simulink model "NonLinearModelPID_DT"  (R2018b)
settings: Solver=VariableStepAuto  StartTime=0.0  StopTime=50  RelTol=1e-3
undefined symbols (not defined in the file): DiscIntNeverNeededParam, Gxd_A_obs, Gxd_B_obs, Gxd_C_obs, Gyawd_A_obs, Gyawd_B_obs, Gyawd_C_obs, Gyd_A_obs, Gyd_B_obs, Gyd_C_obs, Gzd_A_obs, Gzd_B_obs, Gzd_C_obs, K0_X, K0_Y, K0_yaw, K0_Z, K_X, K_Y, K_yaw, K_Z, KGe_X, KGe_Y, KGe_yaw, KGe_Z, t_samp
libraries: simulink x5
settings Model: Creator=Henrique  LastModifiedBy=Henrique

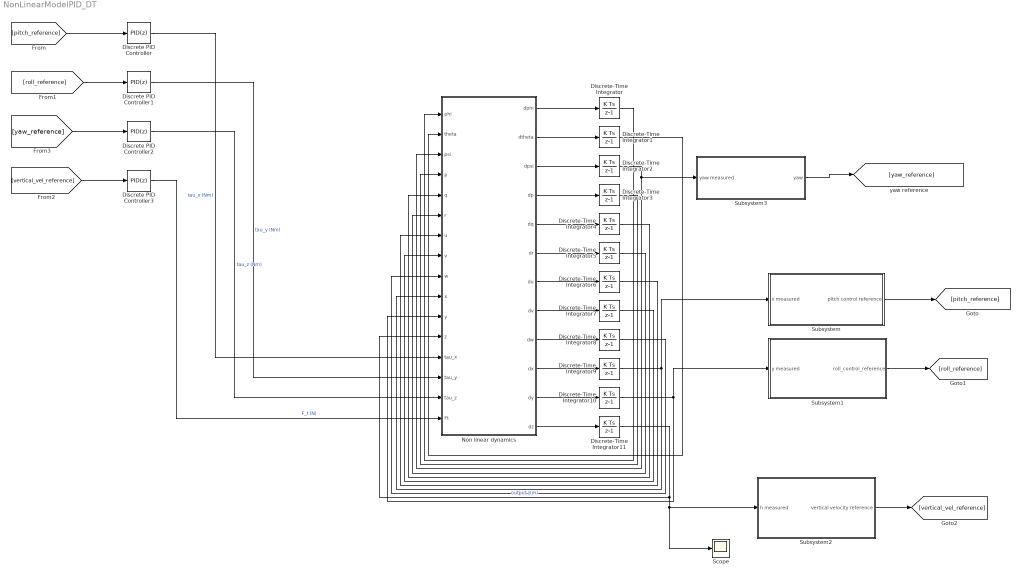
== system NonLinearModelPID_DT ==
  Discrete PID Controller : simulink/Continuous/PID Controller  Controller=PID  Form=Parallel  TimeDomain=Discrete-time  SampleTime=-1  IntegratorMethod=Forward Euler  FilterMethod=Forward Euler  ControllerParametersSource=internal  P=-0.0333564660904056  I=-0.00367562518786493  D=0.0674784843331279  UseFilter=on  N=0.484796452160315  TunerSelectOption=Transfer Function Based (PID Tuner App)  InitialConditionSource=internal  InitialConditionForIntegrator=0  InitialConditionForFilter=0  DifferentiatorICPrevScaledInput=0  ExternalReset=none  TrackingMode=off  Kt=1  LimitOutput=off  UpperSaturationLimit=inf  LowerSaturationLimit=-inf  LinearizeAsGain=off  AntiWindupMode=none  Kb=1  POutMin=[]  POutMax=[]  IOutMin=[]  IOutMax=[]  DOutMin=[]  DOutMax=[]  NOutMin=[]  NOutMax=[]  SumOutMin=[]  SumOutMax=[]  SaturationOutMin=[]  SaturationOutMax=[]  PParamMin=[]  PParamMax=[]  IParamMin=[]  IParamMax=[]  DParamMin=[]  DParamMax=[]  NParamMin=[]  NParamMax=[]  KbParamMin=[]  KbParamMax=[]  KtParamMin=[]  KtParamMax=[]  KbOutMin=[]  KbOutMax=[]  KtOutMin=[]  KtOutMax=[]  IntegratorOutMin=[]  IntegratorOutMax=[]  FilterOutMin=[]  FilterOutMax=[]  SumI1OutMin=[]  SumI1OutMax=[]  SumI2OutMin=[]  SumI2OutMax=[]  SumI3OutMin=[]  SumI3OutMax=[]  SumI4OutMin=[]  SumI4OutMax=[]  SumDOutMin=[]  SumDOutMax=[]  DifferentiatorOutMin=[]  DifferentiatorOutMax=[]  FilterDiffOutCoefMin=[]  FilterDiffOutCoefMax=[]  ReciprocalOutMin=[]  ReciprocalOutMax=[]  SumDenOutMin=[]  SumDenOutMax=[]  SumNumOutMin=[]  SumNumOutMax=[]  DivideOutMin=[]  DivideOutMax=[]  IntegratorContinuousStateAttributes=''  IntegratorStateMustResolveToSignalObject=off  IntegratorRTWStateStorageClass=Auto  FilterContinuousStateAttributes=''  FilterStateMustResolveToSignalObject=off  FilterRTWStateStorageClass=Auto  ParallelPVariant=InternalParameters  IdealPVariant=Disabled  IVariant=InternalParameters  DVariant=InternalParameters  IntegratorVariant=Discrete  SatVariant=Disabled  AWVariant=Passthrough  PCopyVariant=Disabled  TRVariant=Disabled  FdbkBlocksVariant=Forward  IdealPFdbkVariant=Disabled  SatFdbkVariant=Disabled  DerivativeFilterVariant=ForwardEulerFilter  NVariant=InternalParameters  NCopyVariant=Disabled  FilterICVariant=InternalICsFilter  IntegratorICVariant=InternalICs  ExternalResetVariant=Disabled  TRSumVariant=Passthrough  SumFdbkVariant=Disabled  SumVariant=Sum_PID
  Discrete PID Controller1 : simulink/Continuous/PID Controller  Controller=PID  Form=Parallel  TimeDomain=Discrete-time  SampleTime=-1  IntegratorMethod=Forward Euler  FilterMethod=Forward Euler  ControllerParametersSource=internal  P=0  I=-15.3846153846154  D=0  UseFilter=on  N=100  TunerSelectOption=Transfer Function Based (PID Tuner App)  InitialConditionSource=internal  InitialConditionForIntegrator=0  InitialConditionForFilter=0  DifferentiatorICPrevScaledInput=0  ExternalReset=none  TrackingMode=off  Kt=1  LimitOutput=off  UpperSaturationLimit=inf  LowerSaturationLimit=-inf  LinearizeAsGain=off  AntiWindupMode=none  Kb=1  POutMin=[]  POutMax=[]  IOutMin=[]  IOutMax=[]  DOutMin=[]  DOutMax=[]  NOutMin=[]  NOutMax=[]  SumOutMin=[]  SumOutMax=[]  SaturationOutMin=[]  SaturationOutMax=[]  PParamMin=[]  PParamMax=[]  IParamMin=[]  IParamMax=[]  DParamMin=[]  DParamMax=[]  NParamMin=[]  NParamMax=[]  KbParamMin=[]  KbParamMax=[]  KtParamMin=[]  KtParamMax=[]  KbOutMin=[]  KbOutMax=[]  KtOutMin=[]  KtOutMax=[]  IntegratorOutMin=[]  IntegratorOutMax=[]  FilterOutMin=[]  FilterOutMax=[]  SumI1OutMin=[]  SumI1OutMax=[]  SumI2OutMin=[]  SumI2OutMax=[]  SumI3OutMin=[]  SumI3OutMax=[]  SumI4OutMin=[]  SumI4OutMax=[]  SumDOutMin=[]  SumDOutMax=[]  DifferentiatorOutMin=[]  DifferentiatorOutMax=[]  FilterDiffOutCoefMin=[]  FilterDiffOutCoefMax=[]  ReciprocalOutMin=[]  ReciprocalOutMax=[]  SumDenOutMin=[]  SumDenOutMax=[]  SumNumOutMin=[]  SumNumOutMax=[]  DivideOutMin=[]  DivideOutMax=[]  IntegratorContinuousStateAttributes=''  IntegratorStateMustResolveToSignalObject=off  IntegratorRTWStateStorageClass=Auto  FilterContinuousStateAttributes=''  FilterStateMustResolveToSignalObject=off  FilterRTWStateStorageClass=Auto  ParallelPVariant=InternalParameters  IdealPVariant=Disabled  IVariant=InternalParameters  DVariant=InternalParameters  IntegratorVariant=Discrete  SatVariant=Disabled  AWVariant=Passthrough  PCopyVariant=Disabled  TRVariant=Disabled  FdbkBlocksVariant=Forward  IdealPFdbkVariant=Disabled  SatFdbkVariant=Disabled  DerivativeFilterVariant=ForwardEulerFilter  NVariant=InternalParameters  NCopyVariant=Disabled  FilterICVariant=InternalICsFilter  IntegratorICVariant=InternalICs  ExternalResetVariant=Disabled  TRSumVariant=Passthrough  SumFdbkVariant=Disabled  SumVariant=Sum_PID
  Discrete PID Controller2 : simulink/Continuous/PID Controller  Controller=PID  Form=Parallel  TimeDomain=Discrete-time  SampleTime=-1  IntegratorMethod=Forward Euler  FilterMethod=Forward Euler  ControllerParametersSource=internal  P=0.543386875523055  I=0.00238070680971624  D=-18.3910670245527  UseFilter=on  N=0.0295136960787654  TunerSelectOption=Transfer Function Based (PID Tuner App)  InitialConditionSource=internal  InitialConditionForIntegrator=0  InitialConditionForFilter=0  DifferentiatorICPrevScaledInput=0  ExternalReset=none  TrackingMode=off  Kt=1  LimitOutput=off  UpperSaturationLimit=inf  LowerSaturationLimit=-inf  LinearizeAsGain=off  AntiWindupMode=none  Kb=1  POutMin=[]  POutMax=[]  IOutMin=[]  IOutMax=[]  DOutMin=[]  DOutMax=[]  NOutMin=[]  NOutMax=[]  SumOutMin=[]  SumOutMax=[]  SaturationOutMin=[]  SaturationOutMax=[]  PParamMin=[]  PParamMax=[]  IParamMin=[]  IParamMax=[]  DParamMin=[]  DParamMax=[]  NParamMin=[]  NParamMax=[]  KbParamMin=[]  KbParamMax=[]  KtParamMin=[]  KtParamMax=[]  KbOutMin=[]  KbOutMax=[]  KtOutMin=[]  KtOutMax=[]  IntegratorOutMin=[]  IntegratorOutMax=[]  FilterOutMin=[]  FilterOutMax=[]  SumI1OutMin=[]  SumI1OutMax=[]  SumI2OutMin=[]  SumI2OutMax=[]  SumI3OutMin=[]  SumI3OutMax=[]  SumI4OutMin=[]  SumI4OutMax=[]  SumDOutMin=[]  SumDOutMax=[]  DifferentiatorOutMin=[]  DifferentiatorOutMax=[]  FilterDiffOutCoefMin=[]  FilterDiffOutCoefMax=[]  ReciprocalOutMin=[]  ReciprocalOutMax=[]  SumDenOutMin=[]  SumDenOutMax=[]  SumNumOutMin=[]  SumNumOutMax=[]  DivideOutMin=[]  DivideOutMax=[]  IntegratorContinuousStateAttributes=''  IntegratorStateMustResolveToSignalObject=off  IntegratorRTWStateStorageClass=Auto  FilterContinuousStateAttributes=''  FilterStateMustResolveToSignalObject=off  FilterRTWStateStorageClass=Auto  ParallelPVariant=InternalParameters  IdealPVariant=Disabled  IVariant=InternalParameters  DVariant=InternalParameters  IntegratorVariant=Discrete  SatVariant=Disabled  AWVariant=Passthrough  PCopyVariant=Disabled  TRVariant=Disabled  FdbkBlocksVariant=Forward  IdealPFdbkVariant=Disabled  SatFdbkVariant=Disabled  DerivativeFilterVariant=ForwardEulerFilter  NVariant=InternalParameters  NCopyVariant=Disabled  FilterICVariant=InternalICsFilter  IntegratorICVariant=InternalICs  ExternalResetVariant=Disabled  TRSumVariant=Passthrough  SumFdbkVariant=Disabled  SumVariant=Sum_PID
  Discrete PID Controller3 : simulink/Continuous/PID Controller  Controller=PID  Form=Parallel  TimeDomain=Discrete-time  SampleTime=-1  IntegratorMethod=Forward Euler  FilterMethod=Forward Euler  ControllerParametersSource=internal  P=0.976339800048944  I=0.0350960697623535  D=-5.13778024139935  UseFilter=on  N=0.188645718555451  TunerSelectOption=Transfer Function Based (PID Tuner App)  InitialConditionSource=internal  InitialConditionForIntegrator=0  InitialConditionForFilter=0  DifferentiatorICPrevScaledInput=0  ExternalReset=none  TrackingMode=off  Kt=1  LimitOutput=off  UpperSaturationLimit=inf  LowerSaturationLimit=-inf  LinearizeAsGain=off  AntiWindupMode=none  Kb=1  POutMin=[]  POutMax=[]  IOutMin=[]  IOutMax=[]  DOutMin=[]  DOutMax=[]  NOutMin=[]  NOutMax=[]  SumOutMin=[]  SumOutMax=[]  SaturationOutMin=[]  SaturationOutMax=[]  PParamMin=[]  PParamMax=[]  IParamMin=[]  IParamMax=[]  DParamMin=[]  DParamMax=[]  NParamMin=[]  NParamMax=[]  KbParamMin=[]  KbParamMax=[]  KtParamMin=[]  KtParamMax=[]  KbOutMin=[]  KbOutMax=[]  KtOutMin=[]  KtOutMax=[]  IntegratorOutMin=[]  IntegratorOutMax=[]  FilterOutMin=[]  FilterOutMax=[]  SumI1OutMin=[]  SumI1OutMax=[]  SumI2OutMin=[]  SumI2OutMax=[]  SumI3OutMin=[]  SumI3OutMax=[]  SumI4OutMin=[]  SumI4OutMax=[]  SumDOutMin=[]  SumDOutMax=[]  DifferentiatorOutMin=[]  DifferentiatorOutMax=[]  FilterDiffOutCoefMin=[]  FilterDiffOutCoefMax=[]  ReciprocalOutMin=[]  ReciprocalOutMax=[]  SumDenOutMin=[]  SumDenOutMax=[]  SumNumOutMin=[]  SumNumOutMax=[]  DivideOutMin=[]  DivideOutMax=[]  IntegratorContinuousStateAttributes=''  IntegratorStateMustResolveToSignalObject=off  IntegratorRTWStateStorageClass=Auto  FilterContinuousStateAttributes=''  FilterStateMustResolveToSignalObject=off  FilterRTWStateStorageClass=Auto  ParallelPVariant=InternalParameters  IdealPVariant=Disabled  IVariant=InternalParameters  DVariant=InternalParameters  IntegratorVariant=Discrete  SatVariant=Disabled  AWVariant=Passthrough  PCopyVariant=Disabled  TRVariant=Disabled  FdbkBlocksVariant=Forward  IdealPFdbkVariant=Disabled  SatFdbkVariant=Disabled  DerivativeFilterVariant=ForwardEulerFilter  NVariant=InternalParameters  NCopyVariant=Disabled  FilterICVariant=InternalICsFilter  IntegratorICVariant=InternalICs  ExternalResetVariant=Disabled  TRSumVariant=Passthrough  SumFdbkVariant=Disabled  SumVariant=Sum_PID
  Discrete-Time Integrator{,1..11} (12 alike) : DiscreteIntegrator  SampleTime=-1  ICPrevOutput=DiscIntNeverNeededParam  ICPrevScaledInput=DiscIntNeverNeededParam
  "Non linear dynamics " : MATLAB Function  TreatAsAtomicUnit=on
  Scope : Scope
  Subsystem : Subsystem
  Subsystem1 : Subsystem
  Subsystem2 : Subsystem
  Subsystem3 : Subsystem
  wires:
  Discrete PID Controller3/1 -> "Non linear dynamics "/16(Ft)  "F_t (N)"
  Discrete-Time Integrator2/1 -> Subsystem3/1(yaw measured), "Non linear dynamics "/3(psi)
  Discrete PID Controller/1 -> "Non linear dynamics "/13(tau_x)  "tau_x (Nm)"
  [vertical_vel_reference] -> Discrete PID Controller3/1
  [pitch_reference] -> Discrete PID Controller/1
  Discrete PID Controller2/1 -> "Non linear dynamics "/15(tau_z)  "tau_z (Nm)"
  Discrete PID Controller1/1 -> "Non linear dynamics "/14(tau_y)  "tau_y (Nm)"
  Discrete-Time Integrator/1 -> "Non linear dynamics "/1(phi)
  [roll_reference] -> Discrete PID Controller1/1
  Discrete-Time Integrator1/1 -> "Non linear dynamics "/2(theta)
  "Non linear dynamics "/1(dphi) -> Discrete-Time Integrator/1
  "Non linear dynamics "/2(dtheta) -> Discrete-Time Integrator1/1
  "Non linear dynamics "/3(dpsi) -> Discrete-Time Integrator2/1
  "Non linear dynamics "/4(dp) -> Discrete-Time Integrator3/1
  "Non linear dynamics "/5(dq) -> Discrete-Time Integrator4/1
  "Non linear dynamics "/6(dr) -> Discrete-Time Integrator5/1
  "Non linear dynamics "/7(du) -> Discrete-Time Integrator6/1
  "Non linear dynamics "/8(dv) -> Discrete-Time Integrator7/1
  "Non linear dynamics "/11(dy) -> Discrete-Time Integrator10/1
  "Non linear dynamics "/12(dz) -> Discrete-Time Integrator11/1
  Discrete-Time Integrator3/1 -> "Non linear dynamics "/4(p)
  Discrete-Time Integrator4/1 -> "Non linear dynamics "/5(q)
  Discrete-Time Integrator5/1 -> "Non linear dynamics "/6(r)
  Discrete-Time Integrator6/1 -> "Non linear dynamics "/7(u)
  Discrete-Time Integrator7/1 -> "Non linear dynamics "/8(v)
  Discrete-Time Integrator8/1 -> "Non linear dynamics "/9(w)
  Discrete-Time Integrator9/1 -> "Non linear dynamics "/10(x), Subsystem/1(x measured)
  "Non linear dynamics "/9(dw) -> Discrete-Time Integrator8/1
  "Non linear dynamics "/10(dx) -> Discrete-Time Integrator9/1
  Discrete-Time Integrator10/1 -> "Non linear dynamics "/11(y), Subsystem1/1(y measured)
  Discrete-Time Integrator11/1 -> Scope/1, Subsystem2/1(h measured), "Non linear dynamics "/12(z)  "output z(m)"
  Subsystem/1("pitch control reference ") -> [pitch_reference]
  Subsystem1/1("roll_control_reference ") -> [roll_reference]
  Subsystem2/1("vertical velocity reference ") -> [vertical_vel_reference]
  Subsystem3/1("yaw ") -> [yaw_reference]
  [yaw_reference] -> Discrete PID Controller2/1

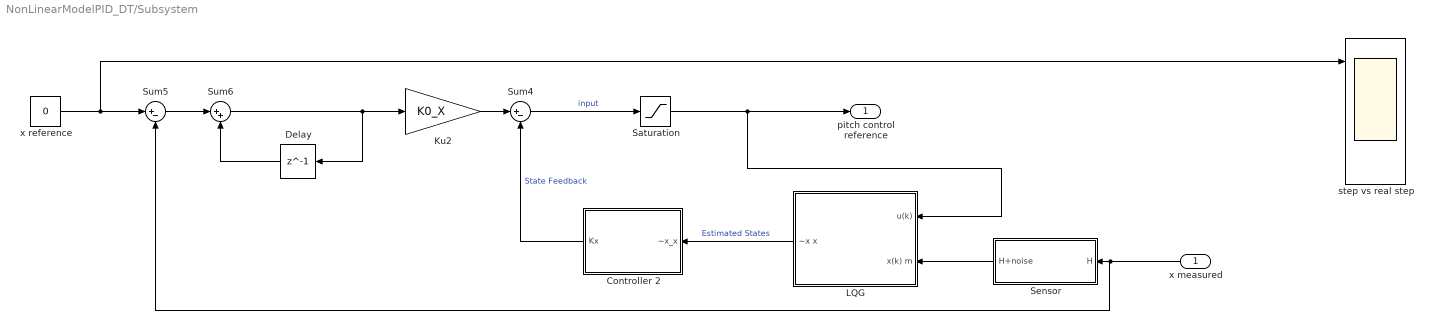
== system NonLinearModelPID_DT/Subsystem ==
  x measured : Inport
  Controller 2 : Subsystem
  Delay : Delay  DelayLength=1  InitialCondition=0
  Ku2 : Gain  Gain=K0_X
  LQG : Subsystem
  Saturation : Saturate  UpperLimit=1  LowerLimit=-1
  Sensor : Subsystem
  Sum4 : Sum  Inputs=|+-
  Sum5 : Sum  Inputs=|+-
  Sum6 : Sum  Inputs=|++
  "step vs real step " : Scope  NumInputPorts=3
  x reference : Constant  Value=0
  "pitch control reference " : Outport
  wires:
  Sum5/1 -> Sum6/1
  Delay/1 -> Sum6/2
  LQG/1("~x x ") -> Controller 2/1(~x_x)  "Estimated States"
  x reference/1 -> Sum5/1, "step vs real step "/1
  Sensor/1(H+noise) -> LQG/2(x(k) m)
  Ku2/1 -> Sum4/1
  Sum6/1 -> Ku2/1, Delay/1
  Controller 2/1(Kx) -> Sum4/2  "State Feedback"
  x measured/1 -> Sum5/2, Sensor/1(H)
  Sum4/1 -> Saturation/1  "input"
  Saturation/1 -> LQG/1(u(k)), "pitch control reference "/1

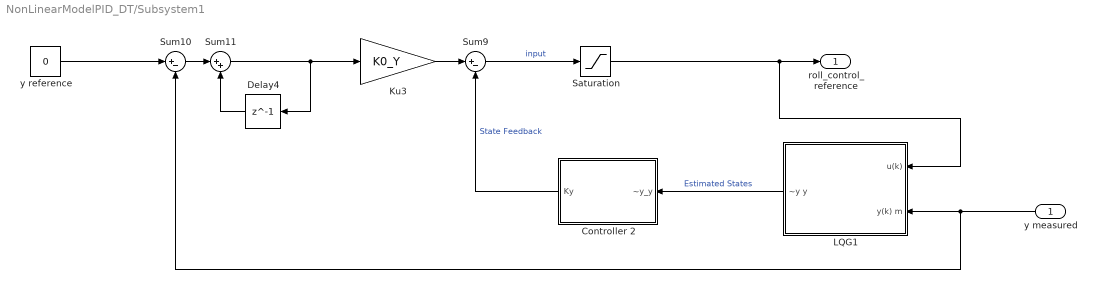
== system NonLinearModelPID_DT/Subsystem1 ==
  y measured : Inport
  Controller 2 : Subsystem
  Delay4 : Delay  DelayLength=1  InitialCondition=0
  Ku3 : Gain  Gain=K0_Y
  LQG1 : Subsystem
  Saturation : Saturate  UpperLimit=1  LowerLimit=-1
  Sum10 : Sum  Inputs=|+-
  Sum11 : Sum  Inputs=|++
  Sum9 : Sum  Inputs=|+-
  y reference : Constant  Value=0
  "roll_control_reference " : Outport
  wires:
  LQG1/1("~y y ") -> Controller 2/1(~y_y)  "Estimated States"
  Sum11/1 -> Delay4/1, Ku3/1
  y reference/1 -> Sum10/1
  Delay4/1 -> Sum11/2
  Sum10/1 -> Sum11/1
  Ku3/1 -> Sum9/1
  y measured/1 -> Sum10/2, LQG1/2(y(k) m)
  Controller 2/1(Ky) -> Sum9/2  "State Feedback"
  Sum9/1 -> Saturation/1  "input"
  Saturation/1 -> LQG1/1(u(k)), "roll_control_reference "/1

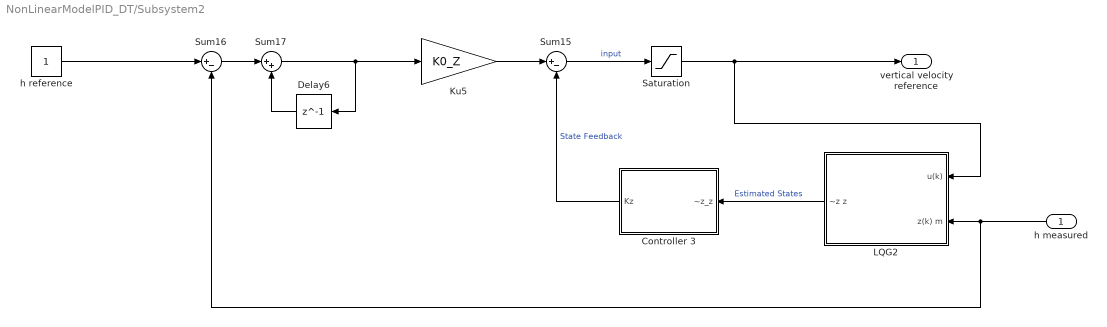
== system NonLinearModelPID_DT/Subsystem2 ==
  h measured : Inport
  Controller 3 : Subsystem
  Delay6 : Delay  DelayLength=1  InitialCondition=0
  Ku5 : Gain  Gain=K0_Z
  LQG2 : Subsystem
  Saturation : Saturate  UpperLimit=1  LowerLimit=-1
  Sum15 : Sum  Inputs=|+-
  Sum16 : Sum  Inputs=|+-
  Sum17 : Sum  Inputs=|++
  h reference : Constant
  "vertical velocity reference " : Outport
  wires:
  Delay6/1 -> Sum17/2
  h measured/1 -> Sum16/2, LQG2/2(z(k) m)
  h reference/1 -> Sum16/1
  LQG2/1("~z z ") -> Controller 3/1(~z_z)  "Estimated States"
  Ku5/1 -> Sum15/1
  Controller 3/1(Kz) -> Sum15/2  "State Feedback"
  Sum17/1 -> Ku5/1, Delay6/1
  Sum16/1 -> Sum17/1
  Sum15/1 -> Saturation/1  "input"
  Saturation/1 -> LQG2/1(u(k)), "vertical velocity reference "/1

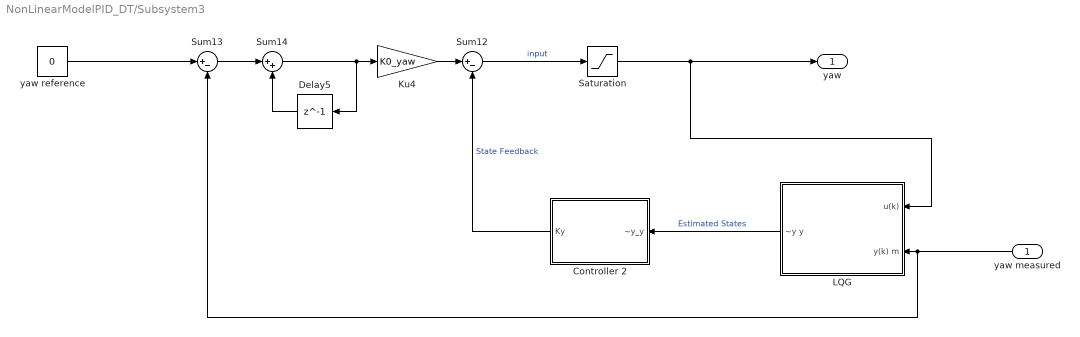
== system NonLinearModelPID_DT/Subsystem3 ==
  yaw measured : Inport
  Controller 2 : Subsystem
  Delay5 : Delay  DelayLength=1  InitialCondition=0
  Ku4 : Gain  Gain=K0_yaw
  "LQG " : Subsystem
  Saturation : Saturate  UpperLimit=1  LowerLimit=-1
  Sum12 : Sum  Inputs=|+-
  Sum13 : Sum  Inputs=|+-
  Sum14 : Sum  Inputs=|++
  yaw reference : Constant  Value=0
  "yaw " : Outport
  wires:
  Sum13/1 -> Sum14/1
  "LQG "/1("~y y ") -> Controller 2/1(~y_y)  "Estimated States"
  Controller 2/1(Ky) -> Sum12/2  "State Feedback"
  yaw measured/1 -> Sum13/2, "LQG "/2(y(k) m)
  Ku4/1 -> Sum12/1
  Sum14/1 -> Delay5/1, Ku4/1
  Delay5/1 -> Sum14/2
  yaw reference/1 -> Sum13/1
  Sum12/1 -> Saturation/1  "input"
  Saturation/1 -> "LQG "/1(u(k)), "yaw "/1

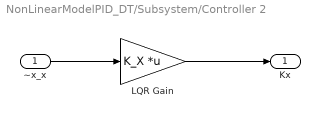
== system NonLinearModelPID_DT/Subsystem/Controller 2 ==
  ~x_x : Inport
  "LQR Gain " : Gain  Gain=K_X  Multiplication=Matrix(K*u) (u vector)
  Kx : Outport
  wires:
  ~x_x/1 -> "LQR Gain "/1
  "LQR Gain "/1 -> Kx/1

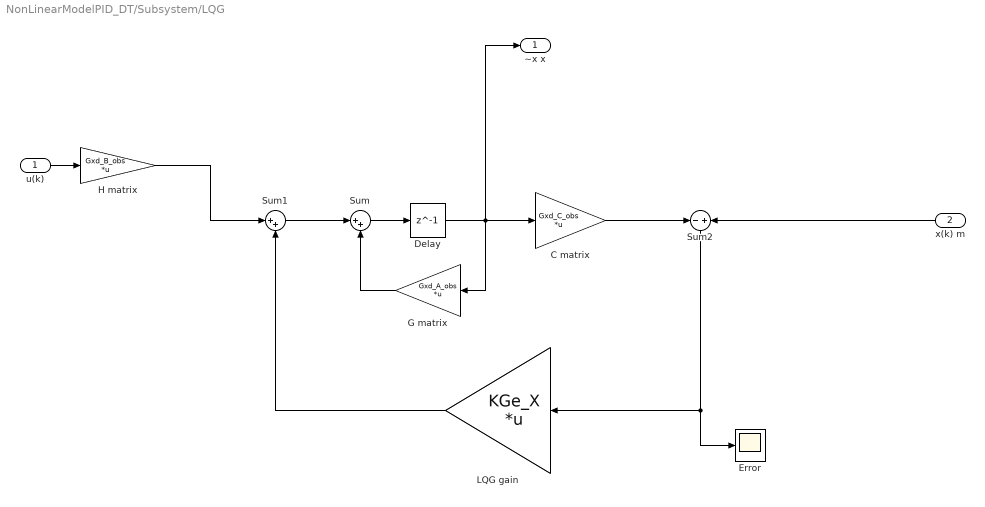
== system NonLinearModelPID_DT/Subsystem/LQG ==
  u(k) : Inport
  x(k) m : Inport  Port=2
  C matrix : Gain  Gain=Gxd_C_obs  Multiplication=Matrix(K*u)
  Delay : Delay  DelayLength=1  InitialCondition=0  SampleTime=t_samp
  Error : Scope
  G matrix : Gain  Gain=Gxd_A_obs  Multiplication=Matrix(K*u)
  H matrix : Gain  Gain=Gxd_B_obs  Multiplication=Matrix(K*u)
  LQG gain : Gain  Gain=KGe_X  Multiplication=Matrix(K*u)
  Sum : Sum  Inputs=|++
  Sum1 : Sum  Inputs=|++
  Sum2 : Sum  Inputs=-+
  "~x x " : Outport
  wires:
  C matrix/1 -> Sum2/1
  x(k) m/1 -> Sum2/2
  H matrix/1 -> Sum1/1
  Sum/1 -> Delay/1
  u(k)/1 -> H matrix/1
  G matrix/1 -> Sum/2
  Sum2/1 -> Error/1, LQG gain/1
  LQG gain/1 -> Sum1/2
  Delay/1 -> "~x x "/1, G matrix/1, C matrix/1
  Sum1/1 -> Sum/1

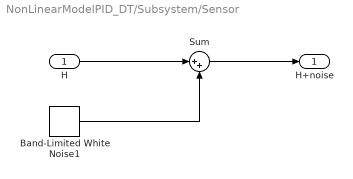
== system NonLinearModelPID_DT/Subsystem/Sensor ==
  H : Inport
  Band-Limited White Noise1 : simulink/Sources/Band-Limited White Noise  Cov=.000001  Ts=0.1  seed=[124123]
  Sum : Sum  Inputs=|++
  H+noise : Outport
  wires:
  Sum/1 -> H+noise/1
  H/1 -> Sum/1
  Band-Limited White Noise1/1 -> Sum/2

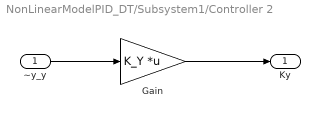
== system NonLinearModelPID_DT/Subsystem1/Controller 2 ==
  ~y_y : Inport
  Gain : Gain  Gain=K_Y  Multiplication=Matrix(K*u) (u vector)
  Ky : Outport
  wires:
  ~y_y/1 -> Gain/1
  Gain/1 -> Ky/1

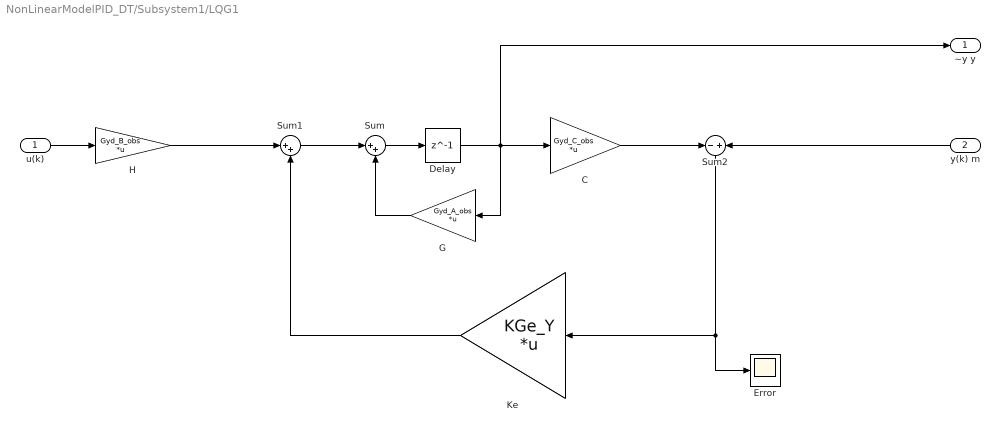
== system NonLinearModelPID_DT/Subsystem1/LQG1 ==
  u(k) : Inport
  y(k) m : Inport  Port=2
  C : Gain  Gain=Gyd_C_obs  Multiplication=Matrix(K*u)
  Delay : Delay  DelayLength=1  InitialCondition=0  SampleTime=t_samp
  Error : Scope
  G : Gain  Gain=Gyd_A_obs  Multiplication=Matrix(K*u)
  H : Gain  Gain=Gyd_B_obs  Multiplication=Matrix(K*u)
  Ke : Gain  Gain=KGe_Y  Multiplication=Matrix(K*u)
  Sum : Sum  Inputs=|++
  Sum1 : Sum  Inputs=|++
  Sum2 : Sum  Inputs=-+
  "~y y " : Outport
  wires:
  C/1 -> Sum2/1
  y(k) m/1 -> Sum2/2
  H/1 -> Sum1/1
  Sum/1 -> Delay/1
  u(k)/1 -> H/1
  G/1 -> Sum/2
  Sum2/1 -> Error/1, Ke/1
  Sum1/1 -> Sum/1
  Ke/1 -> Sum1/2
  Delay/1 -> "~y y "/1, G/1, C/1

== system NonLinearModelPID_DT/Subsystem2/Controller 3 ==
  ~z_z : Inport
  Gain : Gain  Gain=K_Z  Multiplication=Matrix(K*u) (u vector)
  Kz : Outport
  wires:
  ~z_z/1 -> Gain/1
  Gain/1 -> Kz/1

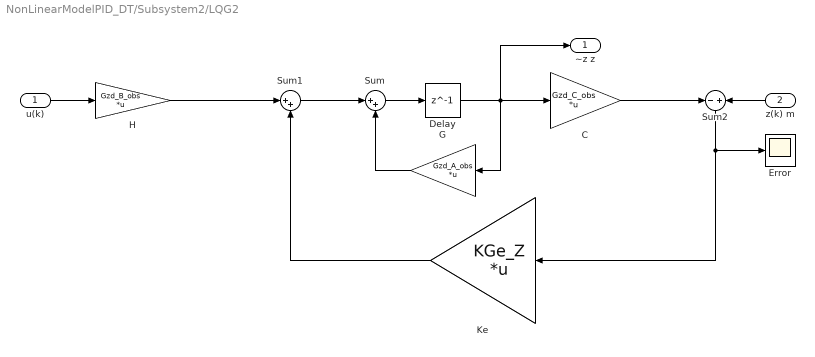
== system NonLinearModelPID_DT/Subsystem2/LQG2 ==
  u(k) : Inport
  z(k) m : Inport  Port=2
  C : Gain  Gain=Gzd_C_obs  Multiplication=Matrix(K*u)
  Delay : Delay  DelayLength=1  InitialCondition=0  SampleTime=t_samp
  Error : Scope
  G : Gain  Gain=Gzd_A_obs  Multiplication=Matrix(K*u)
  H : Gain  Gain=Gzd_B_obs  Multiplication=Matrix(K*u)
  Ke : Gain  Gain=KGe_Z  Multiplication=Matrix(K*u)
  Sum : Sum  Inputs=|++
  Sum1 : Sum  Inputs=|++
  Sum2 : Sum  Inputs=-+
  "~z z " : Outport
  wires:
  C/1 -> Sum2/1
  z(k) m/1 -> Sum2/2
  H/1 -> Sum1/1
  Sum/1 -> Delay/1
  u(k)/1 -> H/1
  G/1 -> Sum/2
  Sum2/1 -> Ke/1, Error/1
  Sum1/1 -> Sum/1
  Ke/1 -> Sum1/2
  Delay/1 -> G/1, "~z z "/1, C/1

== system NonLinearModelPID_DT/Subsystem3/Controller 2 ==
  ~y_y : Inport
  Gain : Gain  Gain=K_yaw  Multiplication=Matrix(K*u) (u vector)
  Ky : Outport
  wires:
  ~y_y/1 -> Gain/1
  Gain/1 -> Ky/1

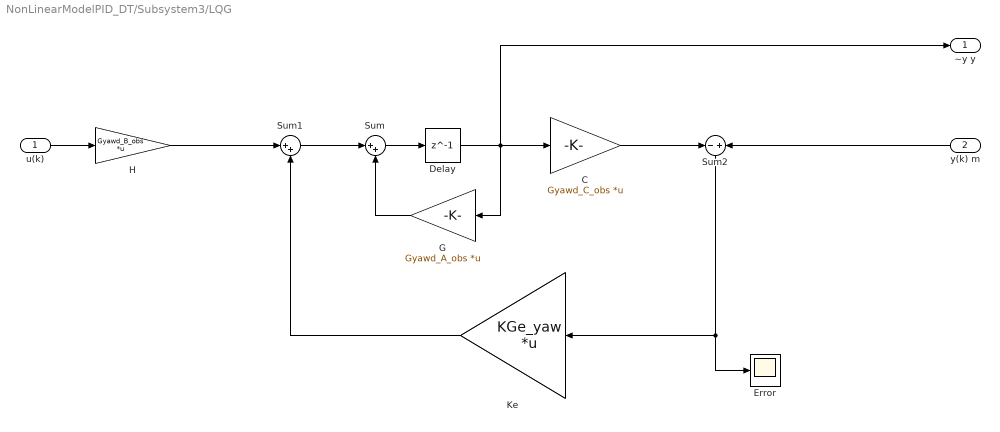
== system NonLinearModelPID_DT/Subsystem3/LQG  ==
  u(k) : Inport
  y(k) m : Inport  Port=2
  C : Gain  Gain=Gyawd_C_obs  Multiplication=Matrix(K*u)
  Delay : Delay  DelayLength=1  InitialCondition=0  SampleTime=t_samp
  Error : Scope
  G : Gain  Gain=Gyawd_A_obs  Multiplication=Matrix(K*u)
  H : Gain  Gain=Gyawd_B_obs  Multiplication=Matrix(K*u)
  Ke : Gain  Gain=KGe_yaw  Multiplication=Matrix(K*u)
  Sum : Sum  Inputs=|++
  Sum1 : Sum  Inputs=|++
  Sum2 : Sum  Inputs=-+
  "~y y " : Outport
  wires:
  C/1 -> Sum2/1
  y(k) m/1 -> Sum2/2
  H/1 -> Sum1/1
  Sum/1 -> Delay/1
  u(k)/1 -> H/1
  G/1 -> Sum/2
  Sum2/1 -> Error/1, Ke/1
  Sum1/1 -> Sum/1
  Ke/1 -> Sum1/2
  Delay/1 -> "~y y "/1, G/1, C/1

== matlab function NonLinearModelPID_DT/Non linear dynamics  ==
  data: phi input size=1; theta input size=1; psi input size=1; p input size=1; q input size=1; r input size=1; u input size=1; dphi output size=1; v input size=1; w input size=1; x input size=1; y input size=1; z input size=1; tau_x input size=1; tau_y input size=1; tau_z input size=1; Ft input size=1; dtheta output size=1; dpsi output size=1; dp output size=1; dq output size=1; dr output size=1; du output size=1; dv output size=1; dw output size=1; dx output size=1; dy output size=1; dz output size=1
%d will represent time derivatives
%wind external forces are neglected
function [dphi,dtheta,dpsi,dp,dq,dr,du,dv,dw,dx,dy,dz] = nonlinear(phi,theta,psi,p,q,r,u,v,w,x,y,z,tau_x,tau_y,tau_z,Ft)
%% parameters
m=0.42; %kg
Ix=0.1;
Iy=0.1;
Iz=0.2;
g=9.81;

%% calculations
dphi=p+r*(cos(phi)*tan(theta))+q*(sin(phi)*tan(theta));
dtheta=q*cos(phi)-r*sin(phi);
dpsi=r*cos(phi)/(cos(theta))+q*sin(phi)/cos(theta);
dp=(Iy-Iz)/Ix*r*q+tau_x/Ix;
dq=(Iz-Ix)/Ix*p*r+tau_y/Iy;
dr=(Ix-Iy)/Iz*p*q+tau_z/Iz;
du=r*v-q*w+g*sin(phi);
dv=p*w-r*u-g*sin(phi)*cos(theta);
dw=q*u-p*v-g*(cos(theta)*cos(phi))+Ft/m;
dx=u*(cos(theta)*cos(psi))+v*(sin(theta)*sin(phi)*cos(psi))+w*(cos(phi)*sin(theta)*cos(psi)+sin(phi)*sin(psi));
dy=u*(cos(theta)*sin(psi))+v*(sin(theta)*sin(phi)*sin(psi)+cos(phi)*cos(psi))+w*(cos(phi)*sin(theta)*sin(psi)-sin(phi)*cos(psi));
dz=u*(-sin(theta))+v*(sin(phi)*cos(theta))+w*(cos(phi)*cos(theta));
end
